simulink model "fig7_41"  (Simulink 4.00)
settings: Solver=ode45  StartTime=0.0  StopTime=5  RelTol=1e-3
settings Model: LastModifiedBy=abbas  LimitDataPoints=off  ExtModeTrigMode=oneshot  ExtModeArmWhenConnect=off  BlockReductionOpt=off

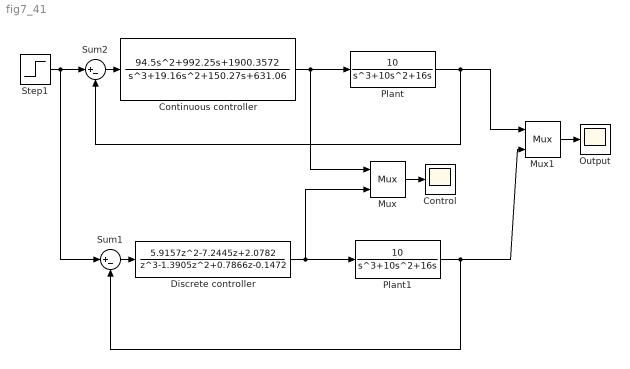
== system fig7_41 ==
  Continuous controller : TransferFcn  Numerator=[94.5 992.25 1900.3572]  Denominator="[1 19.16  150.27 631.06]"  Realization=auto  AbsoluteTolerance=auto
  Control : Scope
      settings: TickLabels=on  TimeRange=auto  YMin=0  YMax=2.75  SaveName=ucd  DataFormat=Array  LimitDataPoints=on  MaxDataPoints=5000
  Discrete controller : DiscreteTransferFcn  Numerator=[5.9157 -7.2445 2.0782]  Denominator=[1 -1.3905 0.7866 -0.1472]  SampleTime=.1  Realization=auto
  Mux : Mux  Inputs=2
      settings: DisplayOption=none
  Mux1 : Mux  Inputs=2
      settings: DisplayOption=none
  Output : Scope
      settings: TickLabels=on  TimeRange=auto  YMin=-5  YMax=5  SaveName=ycd  DataFormat=Array  LimitDataPoints=on  MaxDataPoints=5000
  Plant : TransferFcn  Numerator=[10]  Denominator="[1  10 16 0]"  Realization=auto  AbsoluteTolerance=auto
  Plant1 : TransferFcn  Numerator=[10]  Denominator="[1  10 16 0]"  Realization=auto  AbsoluteTolerance=auto
  Step1 : Step  Time=0  Before=0  After=1  SampleTime=.01
  Sum1 : Sum  Inputs=|+-  SaturateOnIntegerOverflow=off
  Sum2 : Sum  Inputs=|+-  SaturateOnIntegerOverflow=off
  wires:
  Mux/1 -> Control/1
  Mux1/1 -> Output/1
  Sum1/1 -> Discrete controller/1
  Plant/1 -> Mux1/1, Sum2/2
  Sum2/1 -> Continuous controller/1
  Continuous controller/1 -> Plant/1, Mux/1
  Discrete controller/1 -> Plant1/1, Mux/2
  Plant1/1 -> Sum1/2, Mux1/2
  Step1/1 -> Sum2/1, Sum1/1
